simulink model "simu7new"  (R2018b)
settings: Solver=FixedStepAuto  StartTime=0.0  StopTime=100  FixedStep=0.001  RelTol=1e-3
values from neighbouring files (symbols this model uses):
  A1 = k(1)    [Lab6.m]    (also in script7.m = 8; test.m)
  A2 = k(1)    [Lab6.m]    (also in script7.m = 8; test.m)
  Aw1 = 0.1 * k(1)    [Lab6.m]    (also in script7.m = 0.8; test.m)
  Aw2 = 0.1 * k(1)    [Lab6.m]    (also in script7.m = 0.8; test.m)
  dfwe1 = 0    [script7.m]    (also in test.m = 0.2 * fwe1max)
  dfwe2 = 0.1 * fwe2max    [script7.m]    (also in test.m)
  dt = 20    [script7.m]    (also in test.m)
  fwe1 = 0.3 * fwe1max    [script7.m]    (also in test.m = fwe10(i))
  fwe2 = fwe20(i)    [script7.m]    (also in test.m)
  g = 9.81    [Lab6.m]    (also in script7.m; test.m)
  h10 = (fwe1 * fwe1)/(2 * g * Aw1 * Aw1) + h20    [script7.m]    (also in test.m = fwe1^2/(2*Aw1^2*g) + h20)
  h20 = 1/(2 * g * Aw2 * Aw2) * (fwe1 + fwe2) * (fwe1 + fwe2)    [script7.m]    (also in test.m = ((fwe1 + fwe2)^2) / (2*(Aw2^2)*g))
settings Model: Creator=wojciechkonury  LastModifiedBy=wojciechkonury

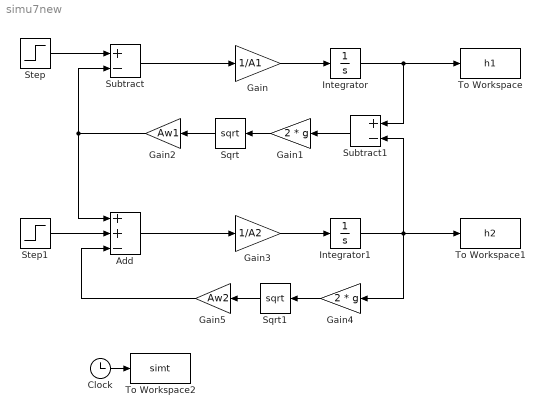
== system simu7new ==
  Add : Sum  Inputs=++-
  Clock : Clock
  Gain : Gain  Gain=1/A1
  Gain1 : Gain  Gain=2 * g
  Gain2 : Gain  Gain=Aw1
  Gain3 : Gain  Gain=1/A2
  Gain4 : Gain  Gain=2 * g
  Gain5 : Gain  Gain=Aw2
  Integrator : Integrator  InitialCondition=h10
  Integrator1 : Integrator  InitialCondition=h20
  Sqrt : Sqrt  SaturateOnIntegerOverflow=on
  Sqrt1 : Sqrt  SaturateOnIntegerOverflow=on
  Step : Step  Time=dt  Before=fwe1  After=fwe1 + dfwe1  SampleTime=0
  Step1 : Step  Time=dt  Before=fwe2  After=fwe2 + dfwe2  SampleTime=0
  Subtract : Sum  Inputs=+-
  Subtract1 : Sum  Inputs=+-
  To Workspace : ToWorkspace  VariableName=h1  SampleTime=-1
  To Workspace1 : ToWorkspace  VariableName=h2  SampleTime=-1
  To Workspace2 : ToWorkspace  VariableName=simt  SampleTime=-1
  wires:
  Step/1 -> Subtract/1
  Subtract/1 -> Gain/1
  Gain/1 -> Integrator/1
  Integrator/1 -> Subtract1/1, To Workspace/1
  Subtract1/1 -> Gain1/1
  Gain1/1 -> Sqrt/1
  Sqrt/1 -> Gain2/1
  Gain2/1 -> Add/1, Subtract/2
  Step1/1 -> Add/2
  Add/1 -> Gain3/1
  Gain3/1 -> Integrator1/1
  Integrator1/1 -> Gain4/1, To Workspace1/1, Subtract1/2
  Sqrt1/1 -> Gain5/1
  Gain4/1 -> Sqrt1/1
  Gain5/1 -> Add/3
  Clock/1 -> To Workspace2/1
